simulink library "HardwareCommunication"  (R2016b)
settings: Solver=VariableStepAuto  StartTime=0.0  StopTime=10.0  RelTol=1e-3
undefined symbols (not defined in the file or in its folder): EthercatDeviceError
libraries: inSOMANET x28, SendToSOMANET x28, VariousLibrary x14, GESHandler x8, InputDeviceHandler x8, PDBHandler x8, SOMANETHandler x8, xpcethercatlib x7, ReceiveFromInputDevice x7, ReceiveFromGES x7, ReceiveFromPDB x7, SendToInputDevice x7
(part 2 of 2)

== system HardwareCommunication/HardwareCommunicationFourJointsInputDevice/ReceivedFourJoints ==
  note: How to do this with EtherCAT, cause they need different inputs.
  Bus Creator10 : BusCreator  Inputs=6  OutDataTypeStr=Bus: EtherCATReceivedFromPDB  NonVirtualBus=on
  Bus Creator{15..18} (4 alike) : BusCreator  Inputs=14  OutDataTypeStr=Bus: EtherCATReceivedFromSOMANET  NonVirtualBus=on
  "EtherCAT Init " : xpcethercatlib/EtherCAT Init   Priority=0  config_file=..\EcatXML\FourJointsWithInputDevice_eni.xml  device_id=0  pci_bus=2  pci_slot=0  dctuning=0  enaDebug=on  enaDC=on  errLink=on  masterDbg=on  stateChgDbg=on  baseClock=off  masterCfg=off  logFile='c:\dbglog.txt'  sample_time=0.002000  DCMode=0
  MuxJointInfo : VariousLibrary/MuxJointInfo
  ReceiveFromInputDevice : ReceiveFromInputDevice/ReceiveFromInputDevice
  ReceiveFromNoGESv2s : ReceiveFromGES/ReceiveFromNoGESv2s
  ReceiveFromPDB : ReceiveFromPDB/ReceiveFromPDB
  Terminator : Terminator
  inSOMANET_LHFE : inSOMANET/inSOMANET_LHFE
  inSOMANET_LKFE : inSOMANET/inSOMANET_LKFE
  inSOMANET_RHFE : inSOMANET/inSOMANET_RHFE
  inSOMANET_RKFE : inSOMANET/inSOMANET_RKFE
  receivedFromSOMANETs : Outport  OutDataTypeStr=Bus: EtherCATReceivedFromSOMANET  PortDimensions=[ 1 4 ]  BusOutputAsStruct=on
  receivedFromInputDevice : Outport  Port=2  OutDataTypeStr=Bus: EtherCATReceivedFromInputDevice  BusOutputAsStruct=on
  receivedFromGESs : Outport  Port=3  OutDataTypeStr=Bus: EtherCATReceivedFromGES  PortDimensions=[1 4]  BusOutputAsStruct=on
  receivedFromPDB : Outport  Port=4  OutDataTypeStr=Bus: EtherCATReceivedFromPDB  BusOutputAsStruct=on
  wires:
  ReceiveFromPDB/2 -> Bus Creator10/2  "buttonPressedPDB"
  ReceiveFromPDB/6 -> Bus Creator10/6  "statusVoltageBattery"
  ReceiveFromPDB/5 -> Bus Creator10/5  "statusCurrentBattery"
  ReceiveFromPDB/4 -> Bus Creator10/4  "statusTemperatureDCDC"
  ReceiveFromPDB/3 -> Bus Creator10/3  "errorMessagePDB"
  ReceiveFromNoGESv2s/1 -> receivedFromGESs/1
  inSOMANET_RHFE/14 -> Bus Creator16/14  "actualMotorVelocity"
  inSOMANET_RHFE/13 -> Bus Creator16/13  "actualMotorAngle"
  inSOMANET_RKFE/14 -> Bus Creator18/14  "actualMotorVelocity"
  inSOMANET_RKFE/13 -> Bus Creator18/13  "actualMotorAngle"
  inSOMANET_LKFE/14 -> Bus Creator17/14  "actualMotorVelocity"
  inSOMANET_LKFE/13 -> Bus Creator17/13  "actualMotorAngle"
  inSOMANET_LHFE/14 -> Bus Creator15/14  "actualMotorVelocity"
  inSOMANET_LHFE/13 -> Bus Creator15/13  "actualMotorAngle"
  "EtherCAT Init "/1 -> Terminator/1
  inSOMANET_LHFE/5 -> Bus Creator15/5  "userMISO"
  Bus Creator10/1 -> receivedFromPDB/1  "receivedFromPDB"
  inSOMANET_LHFE/6 -> Bus Creator15/6  "tuningStatus"
  inSOMANET_LHFE/10 -> Bus Creator15/10  "opMode"
  inSOMANET_LHFE/1 -> Bus Creator15/1  "statusword"
  inSOMANET_LHFE/11 -> Bus Creator15/11  "statusTemperature"
  inSOMANET_RHFE/2 -> Bus Creator16/2  "actualAngle"
  inSOMANET_RHFE/3 -> Bus Creator16/3  "actualVelocity"
  inSOMANET_RHFE/4 -> Bus Creator16/4  "actualTorque"
  inSOMANET_RHFE/6 -> Bus Creator16/6  "tuningStatus"
  inSOMANET_LHFE/2 -> Bus Creator15/2  "actualAngle"
  inSOMANET_RHFE/1 -> Bus Creator16/1  "statusword"
  inSOMANET_RHFE/7 -> Bus Creator16/7  "errorSOMANET"
  inSOMANET_RHFE/9 -> Bus Creator16/9  "statusPhaseCurrentC"
  inSOMANET_RHFE/10 -> Bus Creator16/10  "opMode"
  inSOMANET_LHFE/7 -> Bus Creator15/7  "errorSOMANET"
  inSOMANET_RHFE/11 -> Bus Creator16/11  "statusTemperature"
  Bus Creator15/1 -> [receivedFromLHFE]
  Bus Creator16/1 -> [receivedFromRHFE]
  inSOMANET_LKFE/1 -> Bus Creator17/1  "statusword"
  inSOMANET_LHFE/3 -> Bus Creator15/3  "actualVelocity"
  inSOMANET_RHFE/12 -> Bus Creator16/12  "timestamp"
  inSOMANET_LKFE/2 -> Bus Creator17/2  "actualAngle"
  inSOMANET_LHFE/12 -> Bus Creator15/12  "timestamp"
  inSOMANET_LHFE/4 -> Bus Creator15/4  "actualTorque"
  inSOMANET_LHFE/8 -> Bus Creator15/8  "statusPhaseCurrentB"
  inSOMANET_RHFE/5 -> Bus Creator16/5  "userMISO"
  inSOMANET_RHFE/8 -> Bus Creator16/8  "statusPhaseCurrentB"
  inSOMANET_LKFE/3 -> Bus Creator17/3  "actualVelocity"
  MuxJointInfo/1 -> receivedFromSOMANETs/1
  inSOMANET_LKFE/4 -> Bus Creator17/4  "actualTorque"
  inSOMANET_LKFE/7 -> Bus Creator17/7  "errorSOMANET"
  inSOMANET_LHFE/9 -> Bus Creator15/9  "statusPhaseCurrentC"
  inSOMANET_LKFE/9 -> Bus Creator17/9  "statusPhaseCurrentC"
  inSOMANET_RKFE/4 -> Bus Creator18/4  "actualTorque"
  inSOMANET_RKFE/9 -> Bus Creator18/9  "statusPhaseCurrentC"
  inSOMANET_RKFE/2 -> Bus Creator18/2  "actualAngle"
  inSOMANET_LKFE/10 -> Bus Creator17/10  "opMode"
  inSOMANET_LKFE/6 -> Bus Creator17/6  "tuningStatus"
  inSOMANET_RKFE/10 -> Bus Creator18/10  "opMode"
  Bus Creator17/1 -> [receivedFromLKFE]
  inSOMANET_LKFE/12 -> Bus Creator17/12  "timestamp"
  inSOMANET_LKFE/8 -> Bus Creator17/8  "statusPhaseCurrentB"
  inSOMANET_RKFE/5 -> Bus Creator18/5  "userMISO"
  inSOMANET_RKFE/3 -> Bus Creator18/3  "actualVelocity"
  inSOMANET_RKFE/8 -> Bus Creator18/8  "statusPhaseCurrentB"
  inSOMANET_RKFE/7 -> Bus Creator18/7  "errorSOMANET"
  inSOMANET_LKFE/5 -> Bus Creator17/5  "userMISO"
  inSOMANET_RKFE/1 -> Bus Creator18/1  "statusword"
  inSOMANET_RKFE/6 -> Bus Creator18/6  "tuningStatus"
  inSOMANET_RKFE/12 -> Bus Creator18/12  "timestamp"
  inSOMANET_LKFE/11 -> Bus Creator17/11  "statusTemperature"
  inSOMANET_RKFE/11 -> Bus Creator18/11  "statusTemperature"
  Bus Creator18/1 -> [receivedFromRKFE]
  [receivedFromLHFE] -> MuxJointInfo/1
  [receivedFromRHFE] -> MuxJointInfo/3
  [receivedFromRKFE] -> MuxJointInfo/4
  [receivedFromLKFE] -> MuxJointInfo/2
  ReceiveFromPDB/1 -> Bus Creator10/1  "timestamp"
  ReceiveFromInputDevice/1 -> receivedFromInputDevice/1  "desiredState"

== system HardwareCommunication/HardwareCommunicationFourJointsInputDevice/SendFourJoints ==
  sendToSOMANETs : Inport  OutDataTypeStr=Bus: EtherCATSendToSOMANET  PortDimensions=[1 4]  BusOutputAsStruct=on
  sendToInputDevice : Inport  Port=2  OutDataTypeStr=Bus: EtherCATSendToInputDevice  BusOutputAsStruct=on
  sendToPDB : Inport  Port=3  OutDataTypeStr=Bus: EtherCATSendToPDB  BusOutputAsStruct=on
  Bus Selector10 : BusSelector  OutputSignals=masterState,errorMessage
  DemuxJointInfo : VariousLibrary/DemuxJointInfo
  SendToInputDevice : SendToInputDevice/SendToInputDevice
  SendToPDB : SendToPDB/SendToPDB
  SendToSomanetLHFE : SendToSOMANET/SendToSomanetLHFE
  SendToSomanetLKFE : SendToSOMANET/SendToSomanetLKFE
  SendToSomanetRHFE : SendToSOMANET/SendToSomanetRHFE
  SendToSomanetRKFE : SendToSOMANET/SendToSomanetRKFE
  wires:
  sendToPDB/1 -> SendToPDB/1
  sendToSOMANETs/1 -> DemuxJointInfo/1
  DemuxJointInfo/3 -> SendToSomanetRHFE/1
  DemuxJointInfo/2 -> SendToSomanetLKFE/1
  DemuxJointInfo/1 -> SendToSomanetLHFE/1
  Bus Selector10/2 -> SendToInputDevice/2  "<errorMessage>"
  Bus Selector10/1 -> SendToInputDevice/1  "<masterState>"
  DemuxJointInfo/4 -> SendToSomanetRKFE/1
  sendToInputDevice/1 -> Bus Selector10/1

== system HardwareCommunication/HardwareCommunicationJointV1WithInputDevice/ReceivedOneJointWithInputDevice ==
  note: How to do this with EtherCAT, cause they need different inputs.
  Bus Creator10 : BusCreator  Inputs=6  OutDataTypeStr=Bus: EtherCATReceivedFromPDB  NonVirtualBus=on
  Bus Creator{15..18} (4 alike) : BusCreator  Inputs=14  OutDataTypeStr=Bus: EtherCATReceivedFromSOMANET  NonVirtualBus=on
  "EtherCAT Init " : xpcethercatlib/EtherCAT Init   Priority=0  config_file=D:\Software\Team_16-17\simulink-models\EcatXML\SingleJointNoGESInputDevice_eni.xml  device_id=1  pci_bus=2  pci_slot=0  dctuning=0  enaDebug=off  enaDC=on  errLink=on  masterDbg=on  stateChgDbg=on  baseClock=off  masterCfg=off  logFile='c:\dbglog.txt'  sample_time=0.002000  DCMode=0
  MuxJointInfo : VariousLibrary/MuxJointInfo
  ReceiveFromInputDevice1 : ReceiveFromInputDevice/ReceiveFromInputDevice
  ReceiveFromNoGESv2s : ReceiveFromGES/ReceiveFromNoGESv2s
  ReceiveFromPDB : ReceiveFromPDB/ReceiveFromPDB
  Terminator : Terminator
  receivedSOMANETLHFEOneJoint : inSOMANET/receivedSOMANETLHFEOneJoint
  receivedSOMANETLKFEOneJoint : inSOMANET/receivedSOMANETLKFEOneJoint
  receivedSOMANETRHFEOneJoint : inSOMANET/receivedSOMANETRHFEOneJoint
  receivedSOMANETRKFEOneJoint : inSOMANET/receivedSOMANETRKFEOneJoint
  receivedFromSOMANETs : Outport  OutDataTypeStr=Bus: EtherCATReceivedFromSOMANET  PortDimensions=[ 1 4 ]  BusOutputAsStruct=on
  receivedFromInputDevice : Outport  Port=2  OutDataTypeStr=Bus: EtherCATReceivedFromInputDevice  BusOutputAsStruct=on
  receivedFromGESs : Outport  Port=3  OutDataTypeStr=Bus: EtherCATReceivedFromGES  PortDimensions=[1 3]  BusOutputAsStruct=on
  receivedFromPDB : Outport  Port=4  OutDataTypeStr=Bus: EtherCATReceivedFromPDB  BusOutputAsStruct=on
  wires:
  ReceiveFromPDB/1 -> Bus Creator10/1  "timestamp"
  ReceiveFromPDB/6 -> Bus Creator10/6  "statusVoltageBattery"
  ReceiveFromPDB/5 -> Bus Creator10/5  "statusCurrentBattery"
  ReceiveFromPDB/4 -> Bus Creator10/4  "statusTemperatureDCDC"
  ReceiveFromPDB/3 -> Bus Creator10/3  "errorMessagePDB"
  ReceiveFromPDB/2 -> Bus Creator10/2  "buttonPressedPDB"
  [receivedFromLKFE] -> MuxJointInfo/2
  [receivedFromRKFE] -> MuxJointInfo/4
  [receivedFromRHFE] -> MuxJointInfo/3
  [receivedFromLHFE] -> MuxJointInfo/1
  Bus Creator18/1 -> [receivedFromRKFE]
  receivedSOMANETRKFEOneJoint/11 -> Bus Creator18/11  "statusTemperature"
  receivedSOMANETLKFEOneJoint/11 -> Bus Creator17/11  "statusTemperature"
  receivedSOMANETRKFEOneJoint/12 -> Bus Creator18/12  "timestamp"
  receivedSOMANETRKFEOneJoint/6 -> Bus Creator18/6  "tuningStatus"
  receivedSOMANETRKFEOneJoint/1 -> Bus Creator18/1  "statusword"
  receivedSOMANETLKFEOneJoint/5 -> Bus Creator17/5  "userMISO"
  receivedSOMANETRKFEOneJoint/7 -> Bus Creator18/7  "errorSOMANET"
  receivedSOMANETRKFEOneJoint/8 -> Bus Creator18/8  "statusPhaseCurrentB"
  receivedSOMANETRKFEOneJoint/3 -> Bus Creator18/3  "actualVelocity"
  receivedSOMANETRKFEOneJoint/5 -> Bus Creator18/5  "userMISO"
  receivedSOMANETLKFEOneJoint/8 -> Bus Creator17/8  "statusPhaseCurrentB"
  receivedSOMANETLKFEOneJoint/12 -> Bus Creator17/12  "timestamp"
  Bus Creator17/1 -> [receivedFromLKFE]
  receivedSOMANETRKFEOneJoint/10 -> Bus Creator18/10  "opMode"
  receivedSOMANETLKFEOneJoint/6 -> Bus Creator17/6  "tuningStatus"
  receivedSOMANETLKFEOneJoint/10 -> Bus Creator17/10  "opMode"
  receivedSOMANETRKFEOneJoint/2 -> Bus Creator18/2  "actualAngle"
  receivedSOMANETRKFEOneJoint/9 -> Bus Creator18/9  "statusPhaseCurrentC"
  receivedSOMANETRKFEOneJoint/4 -> Bus Creator18/4  "actualTorque"
  receivedSOMANETLKFEOneJoint/9 -> Bus Creator17/9  "statusPhaseCurrentC"
  receivedSOMANETLHFEOneJoint/9 -> Bus Creator15/9  "statusPhaseCurrentC"
  receivedSOMANETLKFEOneJoint/7 -> Bus Creator17/7  "errorSOMANET"
  receivedSOMANETLKFEOneJoint/4 -> Bus Creator17/4  "actualTorque"
  MuxJointInfo/1 -> receivedFromSOMANETs/1
  receivedSOMANETLKFEOneJoint/3 -> Bus Creator17/3  "actualVelocity"
  receivedSOMANETRHFEOneJoint/8 -> Bus Creator16/8  "statusPhaseCurrentB"
  receivedSOMANETRHFEOneJoint/5 -> Bus Creator16/5  "userMISO"
  receivedSOMANETLHFEOneJoint/8 -> Bus Creator15/8  "statusPhaseCurrentB"
  receivedSOMANETLHFEOneJoint/4 -> Bus Creator15/4  "actualTorque"
  receivedSOMANETLHFEOneJoint/12 -> Bus Creator15/12  "timestamp"
  receivedSOMANETLKFEOneJoint/2 -> Bus Creator17/2  "actualAngle"
  receivedSOMANETRHFEOneJoint/12 -> Bus Creator16/12  "timestamp"
  receivedSOMANETLHFEOneJoint/3 -> Bus Creator15/3  "actualVelocity"
  receivedSOMANETLKFEOneJoint/1 -> Bus Creator17/1  "statusword"
  Bus Creator16/1 -> [receivedFromRHFE]
  Bus Creator15/1 -> [receivedFromLHFE]
  receivedSOMANETRHFEOneJoint/11 -> Bus Creator16/11  "statusTemperature"
  receivedSOMANETLHFEOneJoint/7 -> Bus Creator15/7  "errorSOMANET"
  receivedSOMANETRHFEOneJoint/10 -> Bus Creator16/10  "opMode"
  receivedSOMANETRHFEOneJoint/9 -> Bus Creator16/9  "statusPhaseCurrentC"
  receivedSOMANETRHFEOneJoint/7 -> Bus Creator16/7  "errorSOMANET"
  receivedSOMANETRHFEOneJoint/1 -> Bus Creator16/1  "statusword"
  receivedSOMANETLHFEOneJoint/2 -> Bus Creator15/2  "actualAngle"
  receivedSOMANETRHFEOneJoint/6 -> Bus Creator16/6  "tuningStatus"
  receivedSOMANETRHFEOneJoint/4 -> Bus Creator16/4  "actualTorque"
  receivedSOMANETRHFEOneJoint/3 -> Bus Creator16/3  "actualVelocity"
  receivedSOMANETRHFEOneJoint/2 -> Bus Creator16/2  "actualAngle"
  receivedSOMANETLHFEOneJoint/11 -> Bus Creator15/11  "statusTemperature"
  receivedSOMANETLHFEOneJoint/1 -> Bus Creator15/1  "statusword"
  receivedSOMANETLHFEOneJoint/10 -> Bus Creator15/10  "opMode"
  receivedSOMANETLHFEOneJoint/6 -> Bus Creator15/6  "tuningStatus"
  Bus Creator10/1 -> receivedFromPDB/1  "receivedFromPDB"
  receivedSOMANETLHFEOneJoint/5 -> Bus Creator15/5  "userMISO"
  "EtherCAT Init "/1 -> Terminator/1
  receivedSOMANETLHFEOneJoint/13 -> Bus Creator15/13  "actualMotorAngle"
  receivedSOMANETLHFEOneJoint/14 -> Bus Creator15/14  "actualMotorVelocity"
  receivedSOMANETLKFEOneJoint/13 -> Bus Creator17/13  "actualMotorAngle"
  receivedSOMANETLKFEOneJoint/14 -> Bus Creator17/14  "actualMotorVelocity"
  receivedSOMANETRKFEOneJoint/13 -> Bus Creator18/13  "actualMotorAngle"
  receivedSOMANETRKFEOneJoint/14 -> Bus Creator18/14  "actualMotorVelocity"
  receivedSOMANETRHFEOneJoint/13 -> Bus Creator16/13  "actualMotorAngle"
  receivedSOMANETRHFEOneJoint/14 -> Bus Creator16/14  "actualMotorVelocity"
  ReceiveFromNoGESv2s/1 -> receivedFromGESs/1
  ReceiveFromInputDevice1/1 -> receivedFromInputDevice/1

== system HardwareCommunication/HardwareCommunicationJointV1WithInputDevice/SendOneJointWithInputDevice ==
  sendToSOMANETs : Inport  OutDataTypeStr=Bus: EtherCATSendToSOMANET  PortDimensions=[1 4]  BusOutputAsStruct=on
  sendToInputDevice : Inport  Port=2  OutDataTypeStr=Bus: EtherCATSendToInputDevice  BusOutputAsStruct=on
  sendToPDB : Inport  Port=3  OutDataTypeStr=Bus: EtherCATSendToPDB  BusOutputAsStruct=on
  Bus Selector10 : BusSelector  OutputSignals=masterState,errorMessage
  DemuxJointInfo : VariousLibrary/DemuxJointInfo
  SendSOMANETLHFEOneJoint : SendToSOMANET/SendSOMANETLHFEOneJoint
  SendSOMANETLKFEOneJoint : SendToSOMANET/SendSOMANETLKFEOneJoint
  SendSOMANETRHFEOneJoint : SendToSOMANET/SendSOMANETRHFEOneJoint
  SendSOMANETRKFEOneJoint : SendToSOMANET/SendSOMANETRKFEOneJoint
  SendToInputDevice1 : SendToInputDevice/SendToInputDevice
  SendToPDB : SendToPDB/SendToPDB
  wires:
  sendToSOMANETs/1 -> DemuxJointInfo/1
  DemuxJointInfo/3 -> SendSOMANETRHFEOneJoint/1
  DemuxJointInfo/2 -> SendSOMANETLKFEOneJoint/1
  DemuxJointInfo/1 -> SendSOMANETLHFEOneJoint/1
  Bus Selector10/2 -> SendToInputDevice1/2  "<errorMessage>"
  sendToPDB/1 -> SendToPDB/1
  Bus Selector10/1 -> SendToInputDevice1/1  "<masterState>"
  DemuxJointInfo/4 -> SendSOMANETRKFEOneJoint/1
  sendToInputDevice/1 -> Bus Selector10/1

== system HardwareCommunication/HardwareCommunicationJointV1WithInputDeviceAndBuzzer/ReceivedOneJointWithInputDevice ==
  note: How to do this with EtherCAT, cause they need different inputs.
  Bus Creator10 : BusCreator  Inputs=6  OutDataTypeStr=Bus: EtherCATReceivedFromPDB  NonVirtualBus=on
  Bus Creator{15..18} (4 alike) : BusCreator  Inputs=14  OutDataTypeStr=Bus: EtherCATReceivedFromSOMANET  NonVirtualBus=on
  "EtherCAT Init " : xpcethercatlib/EtherCAT Init   Priority=0  config_file=D:\Software\Team_16-17\simulink-models\EcatXML\SingleJointGESInputDevice_eni.xml  device_id=0  pci_bus=2  pci_slot=0  dctuning=0  enaDebug=off  enaDC=on  errLink=on  masterDbg=on  stateChgDbg=on  baseClock=off  masterCfg=off  logFile='c:\dbglog.txt'  sample_time=0.002000  DCMode=0
  MuxJointInfo : VariousLibrary/MuxJointInfo
  ReceiveFromBackGESv2s : ReceiveFromGES/ReceiveFromBackGESv2s
  ReceiveFromInputDevice1 : ReceiveFromInputDevice/ReceiveFromInputDevice
  ReceiveFromPDB : ReceiveFromPDB/ReceiveFromPDB
  Terminator : Terminator
  receivedSOMANETLHFEOneJoint : inSOMANET/receivedSOMANETLHFEOneJoint
  receivedSOMANETLKFEOneJoint : inSOMANET/receivedSOMANETLKFEOneJoint
  receivedSOMANETRHFEOneJoint : inSOMANET/receivedSOMANETRHFEOneJoint
  receivedSOMANETRKFEOneJoint : inSOMANET/receivedSOMANETRKFEOneJoint
  receivedFromSOMANETs : Outport  OutDataTypeStr=Bus: EtherCATReceivedFromSOMANET  PortDimensions=[ 1 4 ]  BusOutputAsStruct=on
  receivedFromInputDevice : Outport  Port=2  OutDataTypeStr=Bus: EtherCATReceivedFromInputDevice  BusOutputAsStruct=on
  receivedFromGESs : Outport  Port=3  OutDataTypeStr=Bus: EtherCATReceivedFromGES  PortDimensions=[1 3]  BusOutputAsStruct=on
  receivedFromPDB : Outport  Port=4  OutDataTypeStr=Bus: EtherCATReceivedFromPDB  BusOutputAsStruct=on
  wires:
  ReceiveFromInputDevice1/1 -> receivedFromInputDevice/1
  ReceiveFromPDB/1 -> Bus Creator10/1  "timestamp"
  ReceiveFromPDB/6 -> Bus Creator10/6  "statusVoltageBattery"
  ReceiveFromPDB/5 -> Bus Creator10/5  "statusCurrentBattery"
  ReceiveFromPDB/4 -> Bus Creator10/4  "statusTemperatureDCDC"
  ReceiveFromPDB/3 -> Bus Creator10/3  "errorMessagePDB"
  ReceiveFromPDB/2 -> Bus Creator10/2  "buttonPressedPDB"
  [receivedFromLKFE] -> MuxJointInfo/2
  [receivedFromRKFE] -> MuxJointInfo/4
  [receivedFromRHFE] -> MuxJointInfo/3
  [receivedFromLHFE] -> MuxJointInfo/1
  Bus Creator18/1 -> [receivedFromRKFE]
  receivedSOMANETRKFEOneJoint/11 -> Bus Creator18/11  "statusTemperature"
  receivedSOMANETLKFEOneJoint/11 -> Bus Creator17/11  "statusTemperature"
  receivedSOMANETRKFEOneJoint/12 -> Bus Creator18/12  "timestamp"
  receivedSOMANETRKFEOneJoint/6 -> Bus Creator18/6  "tuningStatus"
  receivedSOMANETRKFEOneJoint/1 -> Bus Creator18/1  "statusword"
  receivedSOMANETLKFEOneJoint/5 -> Bus Creator17/5  "userMISO"
  receivedSOMANETRKFEOneJoint/7 -> Bus Creator18/7  "errorSOMANET"
  receivedSOMANETRKFEOneJoint/8 -> Bus Creator18/8  "statusPhaseCurrentB"
  receivedSOMANETRKFEOneJoint/3 -> Bus Creator18/3  "actualVelocity"
  receivedSOMANETRKFEOneJoint/5 -> Bus Creator18/5  "userMISO"
  receivedSOMANETLKFEOneJoint/8 -> Bus Creator17/8  "statusPhaseCurrentB"
  receivedSOMANETLKFEOneJoint/12 -> Bus Creator17/12  "timestamp"
  Bus Creator17/1 -> [receivedFromLKFE]
  receivedSOMANETRKFEOneJoint/10 -> Bus Creator18/10  "opMode"
  receivedSOMANETLKFEOneJoint/6 -> Bus Creator17/6  "tuningStatus"
  receivedSOMANETLKFEOneJoint/10 -> Bus Creator17/10  "opMode"
  receivedSOMANETRKFEOneJoint/2 -> Bus Creator18/2  "actualAngle"
  receivedSOMANETRKFEOneJoint/9 -> Bus Creator18/9  "statusPhaseCurrentC"
  receivedSOMANETRKFEOneJoint/4 -> Bus Creator18/4  "actualTorque"
  receivedSOMANETLKFEOneJoint/9 -> Bus Creator17/9  "statusPhaseCurrentC"
  receivedSOMANETLHFEOneJoint/9 -> Bus Creator15/9  "statusPhaseCurrentC"
  receivedSOMANETLKFEOneJoint/7 -> Bus Creator17/7  "errorSOMANET"
  receivedSOMANETLKFEOneJoint/4 -> Bus Creator17/4  "actualTorque"
  MuxJointInfo/1 -> receivedFromSOMANETs/1
  receivedSOMANETLKFEOneJoint/3 -> Bus Creator17/3  "actualVelocity"
  receivedSOMANETRHFEOneJoint/8 -> Bus Creator16/8  "statusPhaseCurrentB"
  receivedSOMANETRHFEOneJoint/5 -> Bus Creator16/5  "userMISO"
  receivedSOMANETLHFEOneJoint/8 -> Bus Creator15/8  "statusPhaseCurrentB"
  receivedSOMANETLHFEOneJoint/4 -> Bus Creator15/4  "actualTorque"
  receivedSOMANETLHFEOneJoint/12 -> Bus Creator15/12  "timestamp"
  receivedSOMANETLKFEOneJoint/2 -> Bus Creator17/2  "actualAngle"
  receivedSOMANETRHFEOneJoint/12 -> Bus Creator16/12  "timestamp"
  receivedSOMANETLHFEOneJoint/3 -> Bus Creator15/3  "actualVelocity"
  receivedSOMANETLKFEOneJoint/1 -> Bus Creator17/1  "statusword"
  Bus Creator16/1 -> [receivedFromRHFE]
  Bus Creator15/1 -> [receivedFromLHFE]
  receivedSOMANETRHFEOneJoint/11 -> Bus Creator16/11  "statusTemperature"
  receivedSOMANETLHFEOneJoint/7 -> Bus Creator15/7  "errorSOMANET"
  receivedSOMANETRHFEOneJoint/10 -> Bus Creator16/10  "opMode"
  receivedSOMANETRHFEOneJoint/9 -> Bus Creator16/9  "statusPhaseCurrentC"
  receivedSOMANETRHFEOneJoint/7 -> Bus Creator16/7  "errorSOMANET"
  receivedSOMANETRHFEOneJoint/1 -> Bus Creator16/1  "statusword"
  receivedSOMANETLHFEOneJoint/2 -> Bus Creator15/2  "actualAngle"
  receivedSOMANETRHFEOneJoint/6 -> Bus Creator16/6  "tuningStatus"
  receivedSOMANETRHFEOneJoint/4 -> Bus Creator16/4  "actualTorque"
  receivedSOMANETRHFEOneJoint/3 -> Bus Creator16/3  "actualVelocity"
  receivedSOMANETRHFEOneJoint/2 -> Bus Creator16/2  "actualAngle"
  receivedSOMANETLHFEOneJoint/11 -> Bus Creator15/11  "statusTemperature"
  receivedSOMANETLHFEOneJoint/1 -> Bus Creator15/1  "statusword"
  receivedSOMANETLHFEOneJoint/10 -> Bus Creator15/10  "opMode"
  receivedSOMANETLHFEOneJoint/6 -> Bus Creator15/6  "tuningStatus"
  Bus Creator10/1 -> receivedFromPDB/1  "receivedFromPDB"
  receivedSOMANETLHFEOneJoint/5 -> Bus Creator15/5  "userMISO"
  "EtherCAT Init "/1 -> Terminator/1
  receivedSOMANETLHFEOneJoint/13 -> Bus Creator15/13  "actualMotorAngle"
  receivedSOMANETLHFEOneJoint/14 -> Bus Creator15/14  "actualMotorVelocity"
  receivedSOMANETLKFEOneJoint/13 -> Bus Creator17/13  "actualMotorAngle"
  receivedSOMANETLKFEOneJoint/14 -> Bus Creator17/14  "actualMotorVelocity"
  receivedSOMANETRKFEOneJoint/13 -> Bus Creator18/13  "actualMotorAngle"
  receivedSOMANETRKFEOneJoint/14 -> Bus Creator18/14  "actualMotorVelocity"
  receivedSOMANETRHFEOneJoint/13 -> Bus Creator16/13  "actualMotorAngle"
  receivedSOMANETRHFEOneJoint/14 -> Bus Creator16/14  "actualMotorVelocity"
  ReceiveFromBackGESv2s/1 -> receivedFromGESs/1

== system HardwareCommunication/HardwareCommunicationJointV1WithInputDeviceAndBuzzer/SendOneJointWithInputDevice ==
  sendToSOMANETs : Inport  OutDataTypeStr=Bus: EtherCATSendToSOMANET  PortDimensions=[1 4]  BusOutputAsStruct=on
  sendToInputDevice : Inport  Port=2  OutDataTypeStr=Bus: EtherCATSendToInputDevice  BusOutputAsStruct=on
  sendToGES : Inport  Port=3
  sendToPDB : Inport  Port=4  OutDataTypeStr=Bus: EtherCATSendToPDB  BusOutputAsStruct=on
  DemuxJointInfo : VariousLibrary/DemuxJointInfo
  SendSOMANETLHFEOneJoint : SendToSOMANET/SendSOMANETLHFEOneJoint
  SendSOMANETLKFEOneJoint : SendToSOMANET/SendSOMANETLKFEOneJoint
  SendSOMANETRHFEOneJoint : SendToSOMANET/SendSOMANETRHFEOneJoint
  SendSOMANETRKFEOneJoint : SendToSOMANET/SendSOMANETRKFEOneJoint
  SendToGES : SendToGES/sendToGES
  SendToInputDevice1 : SendToInputDevice/SendToInputDevice
  SendToPDB : SendToPDB/SendToPDB
  wires:
  sendToSOMANETs/1 -> DemuxJointInfo/1
  DemuxJointInfo/3 -> SendSOMANETRHFEOneJoint/1
  DemuxJointInfo/2 -> SendSOMANETLKFEOneJoint/1
  DemuxJointInfo/1 -> SendSOMANETLHFEOneJoint/1
  sendToPDB/1 -> SendToPDB/1
  DemuxJointInfo/4 -> SendSOMANETRKFEOneJoint/1
  sendToGES/1 -> SendToGES/1
  sendToInputDevice/1 -> SendToInputDevice1/1

== system HardwareCommunication/HardwareCommunicationOneJoint/ReceivedOneJoint ==
  note: How to do this with EtherCAT, cause they need different inputs.
  Bus Creator10 : BusCreator  Inputs=6  OutDataTypeStr=Bus: EtherCATReceivedFromPDB  NonVirtualBus=on
  Bus Creator{15..18} (4 alike) : BusCreator  Inputs=14  OutDataTypeStr=Bus: EtherCATReceivedFromSOMANET  NonVirtualBus=on
  "EtherCAT Init " : xpcethercatlib/EtherCAT Init   Priority=0  config_file=D:\Software\Team_16-17\simulink-models\EcatXML\SingleJointGesPdb_eni.xml  device_id=0  pci_bus=2  pci_slot=0  dctuning=0  enaDebug=off  enaDC=on  errLink=on  masterDbg=on  stateChgDbg=on  baseClock=off  masterCfg=off  logFile='c:\dbglog.txt'  sample_time=0.002000  DCMode=0
  MuxJointInfo : VariousLibrary/MuxJointInfo
  ReceiveFromBackGESv2s : ReceiveFromGES/ReceiveFromBackGESv2s
  ReceiveFromInputDeviceDummy : ReceiveFromInputDevice/ReceiveFromInputDeviceDummy
  ReceiveFromPDB : ReceiveFromPDB/ReceiveFromPDB
  Terminator : Terminator
  receivedSOMANETLHFEOneJoint : inSOMANET/receivedSOMANETLHFEOneJoint
  receivedSOMANETLKFEOneJoint : inSOMANET/receivedSOMANETLKFEOneJoint
  receivedSOMANETRHFEOneJoint : inSOMANET/receivedSOMANETRHFEOneJoint
  receivedSOMANETRKFEOneJoint : inSOMANET/receivedSOMANETRKFEOneJoint
  receivedFromSOMANETs : Outport  OutDataTypeStr=Bus: EtherCATReceivedFromSOMANET  PortDimensions=[ 1 4 ]  BusOutputAsStruct=on
  receivedFromInputDevice : Outport  Port=2  OutDataTypeStr=Bus: EtherCATReceivedFromInputDevice  BusOutputAsStruct=on
  receivedFromGESs : Outport  Port=3  OutDataTypeStr=Bus: EtherCATReceivedFromGES  PortDimensions=[1 3]  BusOutputAsStruct=on
  receivedFromPDB : Outport  Port=4  OutDataTypeStr=Bus: EtherCATReceivedFromPDB  BusOutputAsStruct=on
  wires:
  ReceiveFromPDB/1 -> Bus Creator10/1  "timestamp"
  ReceiveFromPDB/6 -> Bus Creator10/6  "statusVoltageBattery"
  ReceiveFromPDB/5 -> Bus Creator10/5  "statusCurrentBattery"
  ReceiveFromPDB/4 -> Bus Creator10/4  "statusTemperatureDCDC"
  ReceiveFromPDB/3 -> Bus Creator10/3  "errorMessagePDB"
  ReceiveFromPDB/2 -> Bus Creator10/2  "buttonPressedPDB"
  [receivedFromLKFE] -> MuxJointInfo/2
  [receivedFromRKFE] -> MuxJointInfo/4
  [receivedFromRHFE] -> MuxJointInfo/3
  [receivedFromLHFE] -> MuxJointInfo/1
  Bus Creator18/1 -> [receivedFromRKFE]
  receivedSOMANETRKFEOneJoint/11 -> Bus Creator18/11  "statusTemperature"
  receivedSOMANETLKFEOneJoint/11 -> Bus Creator17/11  "statusTemperature"
  receivedSOMANETRKFEOneJoint/12 -> Bus Creator18/12  "timestamp"
  receivedSOMANETRKFEOneJoint/6 -> Bus Creator18/6  "tuningStatus"
  receivedSOMANETRKFEOneJoint/1 -> Bus Creator18/1  "statusword"
  receivedSOMANETLKFEOneJoint/5 -> Bus Creator17/5  "userMISO"
  receivedSOMANETRKFEOneJoint/7 -> Bus Creator18/7  "errorSOMANET"
  receivedSOMANETRKFEOneJoint/8 -> Bus Creator18/8  "statusPhaseCurrentB"
  receivedSOMANETRKFEOneJoint/3 -> Bus Creator18/3  "actualVelocity"
  receivedSOMANETRKFEOneJoint/5 -> Bus Creator18/5  "userMISO"
  receivedSOMANETLKFEOneJoint/8 -> Bus Creator17/8  "statusPhaseCurrentB"
  receivedSOMANETLKFEOneJoint/12 -> Bus Creator17/12  "timestamp"
  Bus Creator17/1 -> [receivedFromLKFE]
  receivedSOMANETRKFEOneJoint/10 -> Bus Creator18/10  "opMode"
  receivedSOMANETLKFEOneJoint/6 -> Bus Creator17/6  "tuningStatus"
  receivedSOMANETLKFEOneJoint/10 -> Bus Creator17/10  "opMode"
  receivedSOMANETRKFEOneJoint/2 -> Bus Creator18/2  "actualAngle"
  receivedSOMANETRKFEOneJoint/9 -> Bus Creator18/9  "statusPhaseCurrentC"
  receivedSOMANETRKFEOneJoint/4 -> Bus Creator18/4  "actualTorque"
  receivedSOMANETLKFEOneJoint/9 -> Bus Creator17/9  "statusPhaseCurrentC"
  receivedSOMANETLHFEOneJoint/9 -> Bus Creator15/9  "statusPhaseCurrentC"
  receivedSOMANETLKFEOneJoint/7 -> Bus Creator17/7  "errorSOMANET"
  receivedSOMANETLKFEOneJoint/4 -> Bus Creator17/4  "actualTorque"
  MuxJointInfo/1 -> receivedFromSOMANETs/1
  receivedSOMANETLKFEOneJoint/3 -> Bus Creator17/3  "actualVelocity"
  receivedSOMANETRHFEOneJoint/8 -> Bus Creator16/8  "statusPhaseCurrentB"
  receivedSOMANETRHFEOneJoint/5 -> Bus Creator16/5  "userMISO"
  receivedSOMANETLHFEOneJoint/8 -> Bus Creator15/8  "statusPhaseCurrentB"
  receivedSOMANETLHFEOneJoint/4 -> Bus Creator15/4  "actualTorque"
  receivedSOMANETLHFEOneJoint/12 -> Bus Creator15/12  "timestamp"
  receivedSOMANETLKFEOneJoint/2 -> Bus Creator17/2  "actualAngle"
  receivedSOMANETRHFEOneJoint/12 -> Bus Creator16/12  "timestamp"
  receivedSOMANETLHFEOneJoint/3 -> Bus Creator15/3  "actualVelocity"
  receivedSOMANETLKFEOneJoint/1 -> Bus Creator17/1  "statusword"
  Bus Creator16/1 -> [receivedFromRHFE]
  Bus Creator15/1 -> [receivedFromLHFE]
  receivedSOMANETRHFEOneJoint/11 -> Bus Creator16/11  "statusTemperature"
  receivedSOMANETLHFEOneJoint/7 -> Bus Creator15/7  "errorSOMANET"
  receivedSOMANETRHFEOneJoint/10 -> Bus Creator16/10  "opMode"
  receivedSOMANETRHFEOneJoint/9 -> Bus Creator16/9  "statusPhaseCurrentC"
  receivedSOMANETRHFEOneJoint/7 -> Bus Creator16/7  "errorSOMANET"
  receivedSOMANETRHFEOneJoint/1 -> Bus Creator16/1  "statusword"
  receivedSOMANETLHFEOneJoint/2 -> Bus Creator15/2  "actualAngle"
  receivedSOMANETRHFEOneJoint/6 -> Bus Creator16/6  "tuningStatus"
  receivedSOMANETRHFEOneJoint/4 -> Bus Creator16/4  "actualTorque"
  receivedSOMANETRHFEOneJoint/3 -> Bus Creator16/3  "actualVelocity"
  receivedSOMANETRHFEOneJoint/2 -> Bus Creator16/2  "actualAngle"
  receivedSOMANETLHFEOneJoint/11 -> Bus Creator15/11  "statusTemperature"
  receivedSOMANETLHFEOneJoint/1 -> Bus Creator15/1  "statusword"
  receivedSOMANETLHFEOneJoint/10 -> Bus Creator15/10  "opMode"
  receivedSOMANETLHFEOneJoint/6 -> Bus Creator15/6  "tuningStatus"
  Bus Creator10/1 -> receivedFromPDB/1  "receivedFromPDB"
  receivedSOMANETLHFEOneJoint/5 -> Bus Creator15/5  "userMISO"
  "EtherCAT Init "/1 -> Terminator/1
  receivedSOMANETLHFEOneJoint/13 -> Bus Creator15/13  "actualMotorAngle"
  receivedSOMANETLHFEOneJoint/14 -> Bus Creator15/14  "actualMotorVelocity"
  receivedSOMANETLKFEOneJoint/13 -> Bus Creator17/13  "actualMotorAngle"
  receivedSOMANETLKFEOneJoint/14 -> Bus Creator17/14  "actualMotorVelocity"
  receivedSOMANETRKFEOneJoint/13 -> Bus Creator18/13  "actualMotorAngle"
  receivedSOMANETRKFEOneJoint/14 -> Bus Creator18/14  "actualMotorVelocity"
  receivedSOMANETRHFEOneJoint/13 -> Bus Creator16/13  "actualMotorAngle"
  receivedSOMANETRHFEOneJoint/14 -> Bus Creator16/14  "actualMotorVelocity"
  ReceiveFromBackGESv2s/1 -> receivedFromGESs/1
  ReceiveFromInputDeviceDummy/1 -> receivedFromInputDevice/1

== system HardwareCommunication/HardwareCommunicationOneJoint/SendOneJoint ==
  sendToSOMANETs : Inport  OutDataTypeStr=Bus: EtherCATSendToSOMANET  PortDimensions=[1 4]  BusOutputAsStruct=on
  sendToInputDevice : Inport  Port=2  OutDataTypeStr=Bus: EtherCATSendToInputDevice  BusOutputAsStruct=on
  sendToPDB : Inport  Port=3  OutDataTypeStr=Bus: EtherCATSendToPDB  BusOutputAsStruct=on
  sendToGES : Inport  Port=4  BusOutputAsStruct=on
  DemuxJointInfo : VariousLibrary/DemuxJointInfo
  SendSOMANETLHFEOneJoint : SendToSOMANET/SendSOMANETLHFEOneJoint
  SendSOMANETLKFEOneJoint : SendToSOMANET/SendSOMANETLKFEOneJoint
  SendSOMANETRHFEOneJoint : SendToSOMANET/SendSOMANETRHFEOneJoint
  SendSOMANETRKFEOneJoint : SendToSOMANET/SendSOMANETRKFEOneJoint
  "SendToInputDeviceDummy " : SendToInputDevice/SendToInputDeviceDummy 
  SendToPDB : SendToPDB/SendToPDB
  sendToGES1 : SendToGES/sendToGES
  wires:
  sendToGES/1 -> sendToGES1/1
  sendToInputDevice/1 -> "SendToInputDeviceDummy "/1
  DemuxJointInfo/4 -> SendSOMANETRKFEOneJoint/1
  sendToPDB/1 -> SendToPDB/1
  DemuxJointInfo/1 -> SendSOMANETLHFEOneJoint/1
  DemuxJointInfo/2 -> SendSOMANETLKFEOneJoint/1
  DemuxJointInfo/3 -> SendSOMANETRHFEOneJoint/1
  sendToSOMANETs/1 -> DemuxJointInfo/1
